simulink model "Practica3_simulink"  (R2025a)
settings: Solver=VariableStepAuto  StartTime=0.0  StopTime=10.0  RelTol=1e-3
settings Model: Creator=Francisco  LastModifiedBy=Francisco

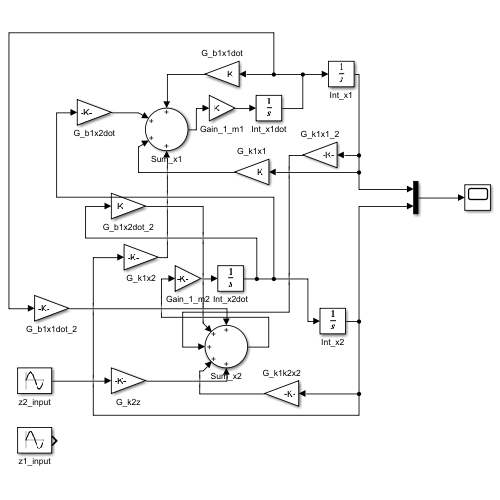
[thumbnail: Simulink's stored preview of the top-level diagram]
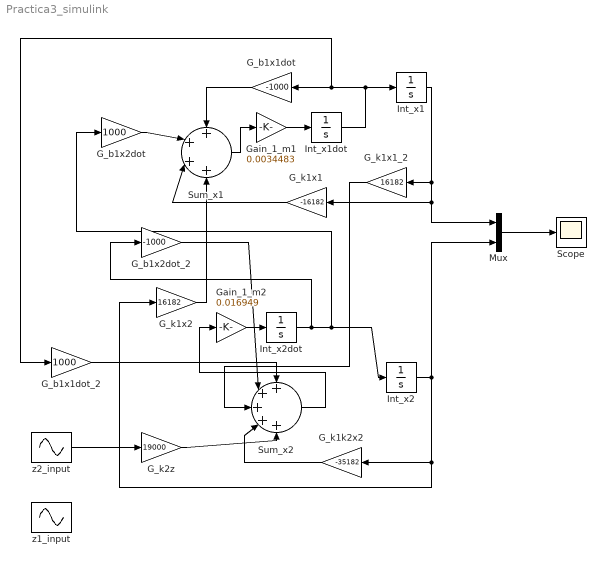
== system Practica3_simulink ==
  G_b1x1dot : Gain  Gain=-1000
  G_b1x1dot_2 : Gain  Gain=1000
  G_b1x2dot : Gain  Gain=1000
  G_b1x2dot_2 : Gain  Gain=-1000
  G_k1k2x2 : Gain  Gain=-35182
  G_k1x1 : Gain  Gain=-16182
  G_k1x1_2 : Gain  Gain=16182
  G_k1x2 : Gain  Gain=16182
  G_k2z : Gain  Gain=19000
  Gain_1_m1 : Gain  Gain=0.0034483
  Gain_1_m2 : Gain  Gain=0.016949
  Int_x1 : Integrator
  Int_x1dot : Integrator
  Int_x2 : Integrator
  Int_x2dot : Integrator
  Mux : Mux  Inputs=2
  Scope : Scope
      settings: ActiveDisplayYMinimum=-0.00810040177813406  ActiveDisplayYMaximum=0.013153484552614714
  Sum_x1 : Sum  Inputs=++++
  Sum_x2 : Sum  Inputs=+++++
  z1_input : Sin  Amplitude=0.05  Frequency=1.5708  SampleTime=0
  z2_input : Sin  Amplitude=0.05  Frequency=62.8319  SampleTime=0
  wires:
  Gain_1_m1/1 -> Int_x1dot/1
  Sum_x1/1 -> Gain_1_m1/1
  G_k1x2/1 -> Sum_x1/4
  G_b1x2dot/1 -> Sum_x1/2
  Int_x2/1 -> G_k1x2/1, G_k1k2x2/1, Mux/2
  Sum_x2/1 -> Gain_1_m2/1
  G_k1k2x2/1 -> Sum_x2/4
  G_k2z/1 -> Sum_x2/5
  Gain_1_m2/1 -> Int_x2dot/1
  G_k1x1_2/1 -> Sum_x2/3
  Int_x2dot/1 -> Int_x2/1, G_b1x2dot/1, G_b1x2dot_2/1
  Mux/1 -> Scope/1
  G_b1x1dot_2/1 -> Sum_x2/1
  G_b1x2dot_2/1 -> Sum_x2/2
  Int_x1/1 -> Mux/1, G_k1x1/1, G_k1x1_2/1
  G_k1x1/1 -> Sum_x1/3
  Int_x1dot/1 -> G_b1x1dot_2/1, G_b1x1dot/1, Int_x1/1
  G_b1x1dot/1 -> Sum_x1/1
  z2_input/1 -> G_k2z/1
